simulink model "RC"  (R2019a)
settings: Solver=VariableStepAuto  StartTime=0.0  StopTime=10.0  RelTol=1e-3
values from neighbouring files (symbols this model uses):
  C = 1    [value.m]
  R = 1    [value.m]
settings Model: Creator=Takumi SHIOTA  LastModifiedBy=Takumi SHIOTA

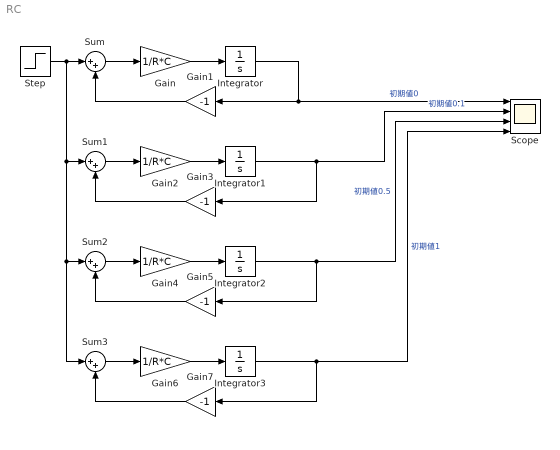
== system RC ==
  Gain{,2,4,6} (4 alike) : Gain  Gain=1/R*C
  Gain{1,3,5,7} (4 alike) : Gain  Gain=-1
  Integrator : Integrator
  Integrator1 : Integrator  InitialCondition=0.1
  Integrator2 : Integrator  InitialCondition=0.5
  Integrator3 : Integrator  InitialCondition=1
  Scope : Scope  NumInputPorts=4
  Step : Step  SampleTime=0
  Sum{,1..3} (4 alike) : Sum  Inputs=|++
  wires:
  Gain1/1 -> Sum/2
  Gain/1 -> Integrator/1
  Step/1 -> Sum3/1, Sum2/1, Sum1/1, Sum/1
  Sum/1 -> Gain/1
  Integrator/1 -> Gain1/1, Scope/1  "初期値0"
  Sum1/1 -> Gain2/1
  Gain2/1 -> Integrator1/1
  Integrator1/1 -> Scope/2, Gain3/1  "初期値0.1"
  Gain3/1 -> Sum1/2
  Gain5/1 -> Sum2/2
  Gain4/1 -> Integrator2/1
  Sum2/1 -> Gain4/1
  Integrator2/1 -> Scope/3, Gain5/1  "初期値0.5"
  Gain7/1 -> Sum3/2
  Gain6/1 -> Integrator3/1
  Sum3/1 -> Gain6/1
  Integrator3/1 -> Scope/4, Gain7/1  "初期値1"
